simulink model "m_SliceSample"  (R2015a)
settings: Solver=FixedStepDiscrete  StartTime=0.0  StopTime=10.0  FixedStep=1  RelTol=1e-3
settings Model: Creator=aohashi  LastModifiedBy=aohashi

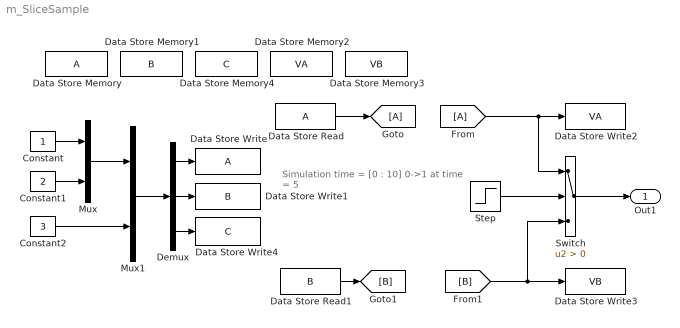
== system m_SliceSample ==
  note: Simulation time = [0 : 10]
      | 0->1 at time = 5
  Constant : Constant
  Constant1 : Constant  Value=2
  Constant2 : Constant  Value=3
  Data Store Memory : DataStoreMemory  ReadBeforeWriteMsg=warning  WriteAfterWriteMsg=warning  WriteAfterReadMsg=warning
  Data Store Memory1 : DataStoreMemory  DataStoreName=B  ReadBeforeWriteMsg=warning  WriteAfterWriteMsg=warning  WriteAfterReadMsg=warning
  Data Store Memory2 : DataStoreMemory  DataStoreName=VA  ReadBeforeWriteMsg=warning  WriteAfterWriteMsg=warning  WriteAfterReadMsg=warning
  Data Store Memory3 : DataStoreMemory  DataStoreName=VB  ReadBeforeWriteMsg=warning  WriteAfterWriteMsg=warning  WriteAfterReadMsg=warning
  Data Store Memory4 : DataStoreMemory  DataStoreName=C  ReadBeforeWriteMsg=warning  WriteAfterWriteMsg=warning  WriteAfterReadMsg=warning
  Data Store Read : DataStoreRead
  Data Store Read1 : DataStoreRead  DataStoreName=B
  Data Store Write : DataStoreWrite
  Data Store Write1 : DataStoreWrite  DataStoreName=B
  Data Store Write2 : DataStoreWrite  DataStoreName=VA
  Data Store Write3 : DataStoreWrite  DataStoreName=VB
  Data Store Write4 : DataStoreWrite  DataStoreName=C
  Demux : Demux  Outputs=3
  Mux : Mux  Inputs=2
  Mux1 : Mux  Inputs=2
  Step : Step  Time=5
  Switch : Switch  Criteria=u2 > Threshold
  Out1 : Outport
  wires:
  Mux/1 -> Mux1/1
  Step/1 -> Switch/2
  Mux1/1 -> Demux/1
  Constant/1 -> Mux/1
  Constant1/1 -> Mux/2
  Constant2/1 -> Mux1/2
  Demux/3 -> Data Store Write4/1
  Demux/1 -> Data Store Write/1
  Demux/2 -> Data Store Write1/1
  Data Store Read/1 -> [A]
  [A] -> Switch/1, Data Store Write2/1
  Switch/1 -> Out1/1
  Data Store Read1/1 -> [B]
  [B] -> Data Store Write3/1, Switch/3
